simulink model "s_ip02_speed_lead"  (Simulink 7.8)
settings: Solver=ode4  StartTime=0.0  StopTime=5  FixedStep=0.002  RelTol=1e-3  AbsTol=1e-6
values from neighbouring files (symbols this model uses):
  a = (1+sin(phi_m)) / (1-sin(phi_m))    [d_ip02_speed_lead.m]
  Kc = db2mag(57)    [d_ip02_speed_lead.m]
  T = 1 / (w_m * sqrt(a))    [d_ip02_speed_lead.m]
undefined symbols (not defined in the file or in its folder): K, tau
settings Model: Creator=Mfotoohi  LastModifiedBy=pmartin  ExtModeTrigDuration=10000  BufferReuse=off
settings SolverCC: PositivePriorityOrder=on
settings DataIOCC: LimitDataPoints=off
settings OptimizationCC: BooleanDataType=off  InlineInvariantSignals=on  OptimizeBlockIOStorage=off  BufferReuse=off  ExpressionFolding=off  FoldNonRolledExpr=off  LocalBlockOutputs=off  InitFltsAndDblsToZero=on
settings DebuggingCC: SaveWithParameterizedLinksMsg=none  SignalResolutionControl=TryResolveAllWithWarning  SolverPrmCheckMsg=none  MultiTaskDSMMsg=warning  MultiTaskCondExecSysMsg=none  FcnCallInpInsideContextMsg=Use local settings  StrictBusMsg=None
settings HardwareCC: TargetHWDeviceType=32-bit Generic
settings RTWCC: SystemTargetFile=quarc_windows.tlc  TemplateMakefile=quarc_default_tmf  Description=Quarc Win32 Target  ProcessScript=quarc_windows_make_rtw_hook  IncludeERTFirstTime=on
settings STFCustomTargetCC: TargetFcnLib=ansi_tfl_tmw.mat  TargetPreCompLibLocation=C:\PROGRA~2\QUARC\lib\2011b\windows\release  SystemTargetFile=quarc_windows.tlc
settings GRTTargetCC: TargetFcnLib=ansi_tfl_tmw.mat  TargetPreCompLibLocation=C:\PROGRA~2\QUARC\lib\2011b\windows\release  ParMdlRefBuildCompliant=off  CompOptLevelCompliant=off  ConcurrentExecutionCompliant=off  MatFileLogging=off  ExtMode=on  ExtModeMexFile=quarc_comm

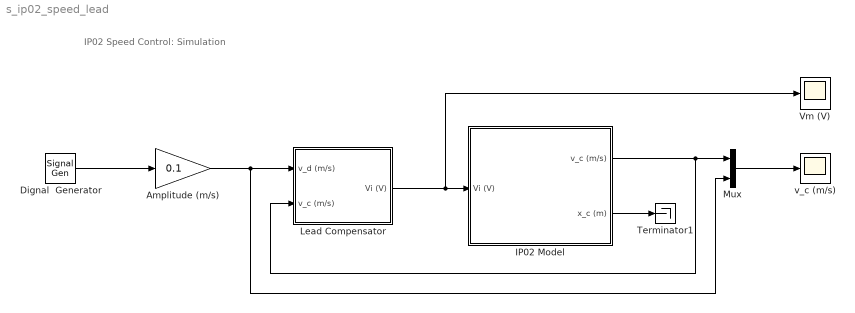
== system s_ip02_speed_lead ==
  note: IP02 Speed Control: Simulation
  Amplitude (m/s) : Gain  Gain=0.1  SaturateOnIntegerOverflow=on  OutDataTypeStr=Inherit: Same as input  ParamDataTypeStr=Inherit: Same as input
  Dignal  Generator : SignalGenerator  WaveForm=square  Frequency=0.5
  IP02 Model : Subsystem
  Lead Compensator : Subsystem
  Mux : Mux  Inputs=2
  Terminator1 : Terminator
  Vm (V) : Scope
      settings: SaveName=data_vm  DataFormat=Array
  v_c (m/s) : Scope
      settings: TickLabels=on  TimeRange=5  YMin=-120  YMax=110  SaveName=data_v  DataFormat=Array
  wires:
  Mux/1 -> v_c (m/s)/1
  Amplitude (m/s)/1 -> Lead Compensator/1(v_d (m/s)), Mux/2
  IP02 Model/1(v_c (m/s)) -> Lead Compensator/2(v_c (m/s)), Mux/1
  IP02 Model/2(x_c (m)) -> Terminator1/1
  Lead Compensator/1(Vi (V)) -> IP02 Model/1(Vi (V)), Vm (V)/1
  Dignal  Generator/1 -> Amplitude (m/s)/1

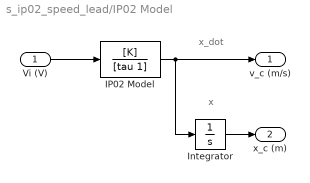
== system s_ip02_speed_lead/IP02 Model ==
  note: x_dot
  note: x
  Vi (V) : Inport
  IP02 Model : TransferFcn  Numerator=[K]  Denominator=[tau 1]
  Integrator : Integrator
  v_c (m/s) : Outport
  x_c (m) : Outport  Port=2
  wires:
  IP02 Model/1 -> v_c (m/s)/1, Integrator/1
  Vi (V)/1 -> IP02 Model/1
  Integrator/1 -> x_c (m)/1

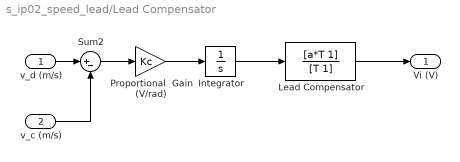
== system s_ip02_speed_lead/Lead Compensator ==
  v_d (m/s) : Inport
  v_c (m/s) : Inport  Port=2
  Integrator : Integrator
  Lead Compensator : TransferFcn  Numerator=[a*T 1]  Denominator=[T 1]
  Proportional  Gain (V/rad) : Gain  Gain=Kc
  Sum2 : Sum  Inputs=|+-
  Vi (V) : Outport
  wires:
  v_c (m/s)/1 -> Sum2/2
  Sum2/1 -> Proportional  Gain (V/rad)/1
  v_d (m/s)/1 -> Sum2/1
  Integrator/1 -> Lead Compensator/1
  Proportional  Gain (V/rad)/1 -> Integrator/1
  Lead Compensator/1 -> Vi (V)/1
